simulink library "TimeSharedLib"  (R2025a)
settings: Solver=VariableStepAuto  StartTime=0.0  StopTime=10.0  RelTol=1e-3
libraries: StdLib x15
settings Model: Creator=peter  LastModifiedBy=peter
settings RTWCC: GPUComputeCapability=3.5

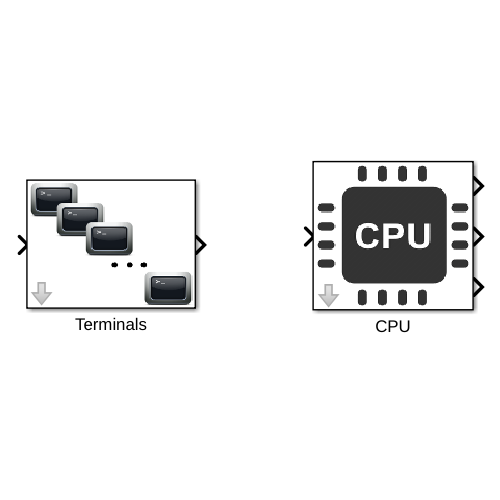
[thumbnail: Simulink's stored preview of the top-level diagram]
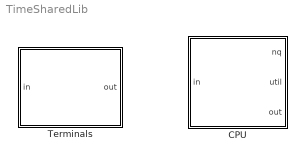
== system TimeSharedLib ==
  CPU : Subsystem  mask{q=0.1, tSwap=0.01}
      mask prompts: q "Time slice"; tSwap "Swap time"
      mask Display: image('$imagefile'); % Use "Edit Image" on toolstrip to change.
  Terminals : Subsystem  mask{N=3, tW=1, tS=1}
      mask prompts: N "Number of terminals"; tW "Waiting time"; tS "Service time"
      mask Display: image('$imagefile'); % Use "Edit Image" on toolstrip to change.

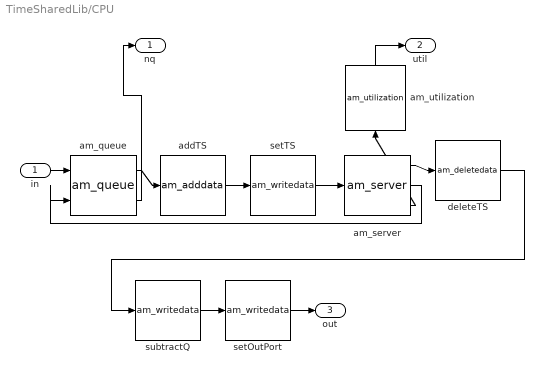
== system TimeSharedLib/CPU ==
  in : Inport
  addTS : StdLib/am_adddata  fields="[\"tSlice\"]"  values="[\"1\"]"  numeric=[true]  infield="\"id\""  tau=[0,0.25]  debug=0
      settings: SourceProductName=Logistics
  am_queue : StdLib/am_queue  tD=[0,2]  tau=[0,1]  debug=0
  am_server : StdLib/am_server  tS=1.0  tsField="\"tSlice\""  tau=[0,1]  debug=0
  am_utilization : StdLib/am_utilization  tau=[0,1]  debug=0
      settings: SourceProductName=Statistics
  deleteTS : StdLib/am_deletedata  fields="\"tSlice\""  tau=[0,0.25]  debug=0
      settings: SourceProductName=Logistics
  setOutPort : StdLib/am_writedata  inFields="[\"remainingServiceTime\"]"  outField="\"outPort\""  changeFunc="\"out = 1 + (in(1) > 0);\""  tau=[0,0.25]  debug=0
      settings: SourceProductName=Logistics
  setTS : StdLib/am_writedata  inFields="[\"remainingServiceTime\"]"  outField="\"tSlice\""  changeFunc="\"out = min(\" + q + \", in(1)) + \" + tSwap + \";\""  tau=[0,0.25]  debug=0
      settings: SourceProductName=Logistics
  subtractQ : StdLib/am_writedata  inFields="[\"remainingServiceTime\"]"  outField="\"remainingServiceTime\""  changeFunc="\"out = max(in(1) - \" + q + \", 0);\""  tau=[0,0.25]  debug=0
      settings: SourceProductName=Logistics
  nq : Outport
  util : Outport  Port=2
  out : Outport  Port=3
  wires:
  in/1 -> am_queue/1
  am_server/1 -> deleteTS/1
  am_queue/2 -> nq/1
  am_server/2 -> am_queue/2
  setTS/1 -> am_server/1
  am_queue/1 -> addTS/1
  addTS/1 -> setTS/1
  deleteTS/1 -> subtractQ/1
  subtractQ/1 -> setOutPort/1
  setOutPort/1 -> out/1
  am_server/3 -> am_utilization/1
  am_utilization/1 -> util/1

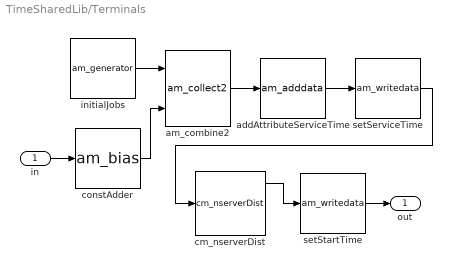
== system TimeSharedLib/Terminals ==
  in : Inport
  addAttributeServiceTime : StdLib/am_adddata  fields="[\"remainingServiceTime\", \"outPort\", \"startTime\"]"  values=[0, 1, 0]  numeric=[true, true, true]  infield="\"id\""  tau=[0,1]  debug=0
      settings: SourceProductName=Logistics
  am_combine2 : StdLib/am_collect2  tD=[0,2]  tau=[0,1]  debug=0
      settings: SourceProductName=Routing
  cm_nserverDist : StdLib/cm_nserverDist  N=N  distName="\"Exponential\""  distPara=[tW]  fieldname="\"waitingTime\""  tD=[0,2]  tau=[0,1]  debug=0
      settings: SourceProductName=Logistics
  constAdder : StdLib/am_bias  bias=N  tau=[0,1]  debug=0
      settings: SourceProductName=Math Operations
  initialJobs : StdLib/am_generator  tG=0  n0=1  nG=N  tD=[0,2]  debug=0
  setServiceTime : StdLib/am_writedata  inFields=[]  outField="\"remainingServiceTime\""  changeFunc="\"out = -\" + tS + \"*log(rand());\""  tau=[0,1]  debug=0
      settings: SourceProductName=Logistics
  setStartTime : StdLib/am_writedata  inFields=[]  outField="\"startTime\""  changeFunc="\"out = get_time();\""  tau=[0,1]  debug=0
      settings: SourceProductName=Logistics
  out : Outport
  wires:
  initialJobs/1 -> am_combine2/1
  am_combine2/1 -> addAttributeServiceTime/1
  addAttributeServiceTime/1 -> setServiceTime/1
  in/1 -> constAdder/1
  constAdder/1 -> am_combine2/2
  setServiceTime/1 -> cm_nserverDist/1
  cm_nserverDist/1 -> setStartTime/1
  setStartTime/1 -> out/1
